simulink model "mppt_power_generation_calculation"  (R2024a)
settings: Solver=VariableStepAuto  StartTime=0.0  StopTime=30  RelTol=1e-3
undefined symbols (not defined in the file): Ion, Lithium
libraries: neural x20, spsSeriesRLCBranchLib x8, spsVoltageMeasurementLib x7, spsDiodeLib x5, spsBreakerLib x4, spsMosfetLib x3, spsBatteryLib x2, spsCurrentMeasurementLib x2, powerlib_extras x2, spsControlledCurrentSourceLib x1, spsPWMGeneratorDCDCLib x1, spsPVArrayLib x1
(part 2 of 2)

== matlab function mppt_power_generation_calculation/Battery Energy Storage System/MATLAB Function ==
  data: currentSoC input; newSoC output; chargeCurrent input; dischargeCurrent input; batteryCapacity input; timeStep input
function newSoC = SoCCalculation(currentSoC, chargeCurrent, dischargeCurrent, batteryCapacity, timeStep)
    % Calculate the new state of charge
    newSoC = currentSoC + (chargeCurrent - dischargeCurrent) * timeStep / (batteryCapacity * 3600); % Convert capacity to Wh
    % Limit the SoC between 0 and 1
    newSoC = max(0, min(0.90, newSoC));
end

== matlab function mppt_power_generation_calculation/Battery Energy Storage System/MATLAB Function1 ==
  data: PVPower input; chargeCurrent output; LoadDemand input; SoC input
function chargeCurrent = chargeControl(PVPower, LoadDemand, SoC)
    maxChargeCurrent = 50; % Maximum charging current in amps
    batteryVoltage = 12; % Example battery voltage
    if SoC < 0.95 % Charge battery if SoC is less than 95%
        excessPower = PVPower - LoadDemand;
        chargeCurrent = min(excessPower / batteryVoltage, maxChargeCurrent); % Adjust based on battery voltage
    else
        chargeCurrent = 0; % Stop charging if SoC >= 95%
    end
end

== matlab function mppt_power_generation_calculation/Battery Energy Storage System/MATLAB Function2 ==
  data: PVPower input; dischargeCurrent output; LoadDemand input; SoC input
function dischargeCurrent = dischargeControl(PVPower, LoadDemand, SoC)
    maxDischargeCurrent = 50; % Maximum discharging current in amps
    batteryVoltage = 12; % Example battery voltage
    if SoC > 0.2 % Discharge battery if SoC is more than 20%
        deficitPower = LoadDemand - PVPower;
        dischargeCurrent = min(deficitPower / batteryVoltage, maxDischargeCurrent); % Adjust based on battery voltage
    else
        dischargeCurrent = 0; % Stop discharging if SoC <= 20%
    end
end

== matlab function mppt_power_generation_calculation/fresnal Algo for irradiance/MATLAB Function ==
  data: S2 input; Ir2 output; Incl input
function Ir2 = optics2(S2, Incl)
    
    %This function computes the reflection, absorption and transmission in
    %the glass to compute the irradiation to the PV cells, the heat absorbed 
    %in the glass and the radiation power absorbed in the PV cells,
    %it is based on Fresnel's laws, depending on the incident angle
    
    Ncell =  72;
    Acell =  0.0225;
    ng = 1.52;
    absg = 0.2;
    dg = 0.01;
    rpv = 0.15;
   

    % Fresnel equations 1st boundary
    r1p =  ( ng^2*cos(Incl) - sqrt(ng^2 - sin(Incl)^2) )^2/( ng^2*cos(Incl) + sqrt( ng^2 - sin(Incl)^2 ) )^2; %P polarization
    r1s =  ( cos(Incl) - sqrt(ng^2 - sin(Incl)^2) )^2/( cos(Incl) + sqrt( ng^2 - sin(Incl)^2 ) )^2; %S polarization
    r1 = 0.5*(r1p + r1s); %Effective reflectance
    t1 = 1-r1;

    nga = 1/ng; %refractive index glass -> air
    th2 = asin(sin(Incl)/ng);  %Snell's law to compute angle of incidence on 2nd boundary

    % Fresnel equations 2nd boundary
    r2p = ( nga^2*cos(th2) - sqrt(nga^2 - sin(th2)^2) )^2/( nga^2*cos(th2) + sqrt( nga^2 - sin(th2)^2 ) )^2 ;
    r2s = ( cos(th2) - sqrt(nga^2 - sin(th2)^2) )^2/( cos(th2) + sqrt( nga^2 - sin(th2)^2 ) )^2 ;
    r2 = 0.5*(r2p + r2s); %Effective reflectance
    t2 = 1 - r2;

    taug = exp(-absg*dg/cos(th2)); 
    
    %Total coefficients for infinite reflections between 2 parallel boundaries
    Transg = t1*taug*t2/(1 - r1*r2*taug^2);
    Reflg = r1 + (t1^2*taug^2*r2)/(1 - r1*r2*taug^2);
    Absg = 1 - Transg - Reflg; 

    Ir2 = S2*Transg; %Irradiation to the PV cells
    heatg = Acell*Ncell*Absg*S2; %heat absorbed in the glass
    powAbspv = Acell*Ncell*Transg*(1-rpv)*S2; %radiation power absorbed by PV cells. Part of it transforms in electrical power
    
end

== matlab function mppt_power_generation_calculation/ ANN solar inputs1/MATLAB Function1 ==
  data: lat input; output output; lon input
function output = generateInput(lat, lon)
    % Get the current date and time
    datetimeNow = datetime('now');
    [~, month, day , hour, ~, ~] = datevec(datetimeNow);

    % Create the output array
    output = [lat; lon; month; day; hour];
end

== matlab function mppt_power_generation_calculation/Subsystem1/battery bank /MATLAB Function ==
  data: SOC input; charge_ctrl output; discharge_ctrl output
function [charge_ctrl, discharge_ctrl] = battery_breaker_control(SOC)
% Inputs:
% SOC  - State of Charge (%)
% Outputs:
% charge_ctrl     - Control signal for the charger (1 = Allow charging, 0 = Stop charging)
% discharge_ctrl  - Control signal for the discharger (1 = Allow discharging, 0 = Stop discharging)

% Define SOC limits
SOC_max = 80; % Maximum SOC limit (%)
SOC_min = 20; % Minimum SOC limit (%)

% Default: Allow charging and discharging
charge_ctrl = 1;    % 1 = Charging allowed
discharge_ctrl = 1; % 1 = Discharging allowed

% Stop charging if SOC exceeds the maximum limit
if SOC > SOC_max
    charge_ctrl = 0; % Stop charging
end

% Stop discharging if SOC drops below the minimum limit
if SOC < SOC_min
    discharge_ctrl = 0; % Stop discharging
end
end
